simulink subsystem "Servomotor_with_resonant_load"  (R2024b)
settings: Solver=VariableStepAuto  StartTime=0.0  StopTime=10.0  RelTol=1e-3
undefined symbols (not defined in the file or in its folder): pulse2deg, sens
settings Model: Creator=Federico Bergami  LastModifiedBy=Federico Bergami

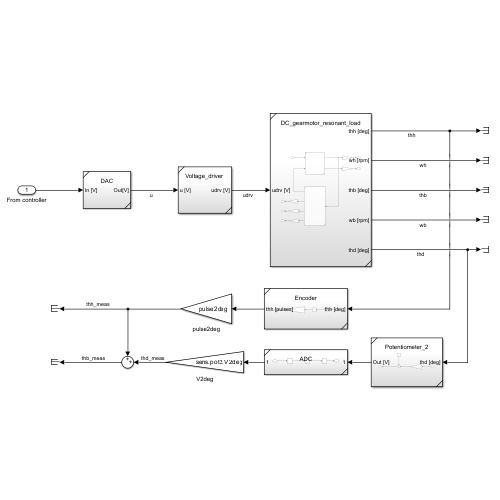
[thumbnail: Simulink's stored preview of the top-level diagram]
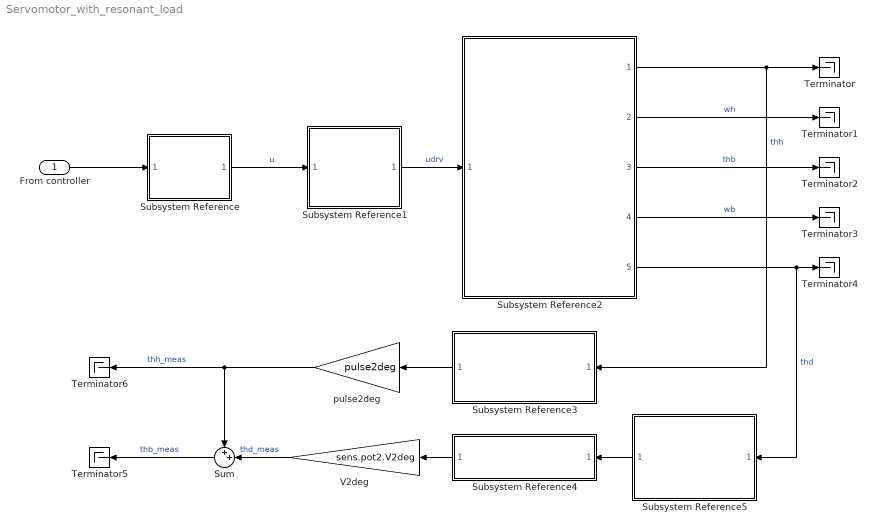
== system Servomotor_with_resonant_load ==
  From controller : Inport
  Subsystem Reference : Subsystem  ReferencedSubsystem=DAC
  Subsystem Reference1 : Subsystem  ReferencedSubsystem=Voltage_driver
  Subsystem Reference2 : Subsystem  ReferencedSubsystem=DC_gearmotor_resonant_load
  Subsystem Reference3 : Subsystem  ReferencedSubsystem=Encoder
  Subsystem Reference4 : Subsystem  ReferencedSubsystem=ADC
  Subsystem Reference5 : Subsystem  ReferencedSubsystem=Potentiometer_2
  Sum : Sum  Inputs=++|
  Terminator{,1..6} (7 alike) : Terminator
  V2deg : Gain  Gain=sens.pot2.V2deg
  pulse2deg : Gain  Gain=pulse2deg
  wires:
  From controller/1 -> Subsystem Reference/1
  Subsystem Reference/1 -> Subsystem Reference1/1  "u"
  Subsystem Reference1/1 -> Subsystem Reference2/1  "udrv"
  Subsystem Reference5/1 -> Subsystem Reference4/1
  Subsystem Reference3/1 -> pulse2deg/1
  Subsystem Reference4/1 -> V2deg/1
  V2deg/1 -> Sum/2  "thd_meas"
  pulse2deg/1 -> Terminator6/1, Sum/1  "thh_meas"
  Subsystem Reference2/2 -> Terminator1/1  "wh"
  Subsystem Reference2/1 -> Subsystem Reference3/1, Terminator/1  "thh"
  Subsystem Reference2/3 -> Terminator2/1  "thb"
  Subsystem Reference2/4 -> Terminator3/1  "wb"
  Subsystem Reference2/5 -> Subsystem Reference5/1, Terminator4/1  "thd"
  Sum/1 -> Terminator5/1  "thb_meas"
